simulink model "SSC17_QuanserPart2_PIDdesign"  (R2016b)
settings: Solver=ode4  StartTime=0.0  StopTime=100  FixedStep=0.01  MaxStep=2.0  RelTol=1e-3  EnableMultiTasking=on
values from neighbouring files (symbols this model uses):
  Kd = G    [UpdatedSimulinkValues-2.m]    (also in UpdatedSimulinkValuesalex1.m; part2a.m = 0.1)
  Ki = G    [UpdatedSimulinkValues-2.m]    (also in UpdatedSimulinkValuesalex1.m; part2a.m = 0.1)
  Kp = G    [UpdatedSimulinkValues-2.m]    (also in UpdatedSimulinkValuesalex1.m; part2a.m = 0.1)
settings Model: Creator=am13440  LastModifiedBy=Alex
settings DataIOCC: LimitDataPoints=on  SaveFormat=Array
settings OptimizationCC: LifeSpan=inf
settings DebuggingCC: UnderspecifiedInitializationDetection=Classic  MergeDetectMultiDrivingBlocksExec=none  SolverPrmCheckMsg=warning  StateNameClashWarn=warning  SFUnexpectedBacktrackingDiag=warning  SFNoUnconditionalDefaultTransitionDiag=warning  SFExecutionAtInitializationDiag=none
settings HardwareCC: ProdBitPerPointer=32  ProdBitPerSizeT=32  ProdBitPerPtrDiffT=32  ProdLargestAtomicFloat=None  ProdIntDivRoundTo=Undefined  ProdEndianess=Unspecified  ProdWordSize=32  ProdHWDeviceType=32-bit Generic
settings ModelReferenceCC: PropagateSignalLabelsOutOfModel=off
settings GRTTargetCC: TargetLangStandard=C89/C90 (ANSI)  GeneratePreprocessorConditionals=Disable all
settings ConfigComp: CovMetricSettings=dw  CovHtmlReporting=on  CovSaveCumulativeToWorkspaceVar=on  CovSaveSingleToWorkspaceVar=on  CovExternalEMLEnable=off  CovSFcnEnable=off

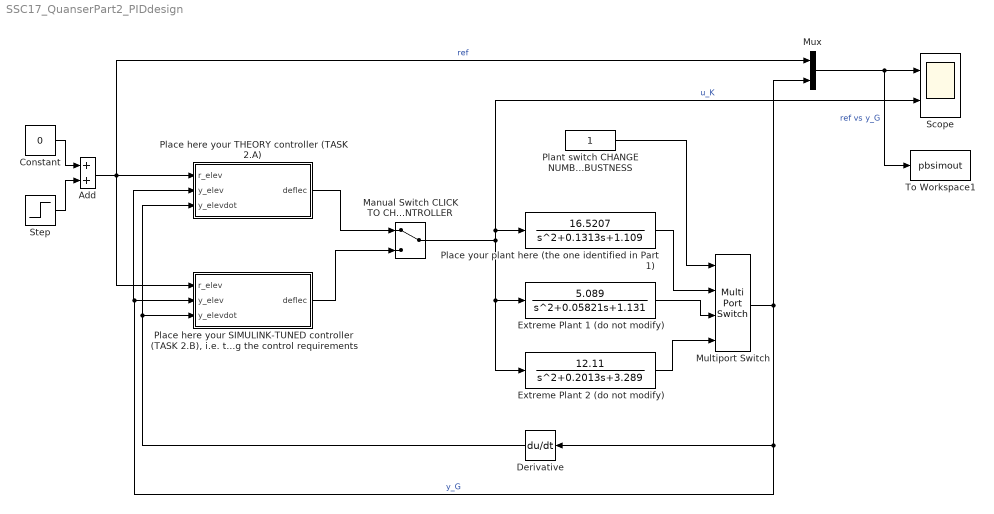
== system SSC17_QuanserPart2_PIDdesign ==
  Add : Sum
  Constant : Constant  Value=0
  Derivative : Derivative  CoefficientInTFapproximation=100
  Extreme Plant 1 (do not modify) : TransferFcn  Numerator=[5.089]  Denominator="[1  0.05821   1.131]"
  Extreme Plant 2 (do not modify) : TransferFcn  Numerator=[12.11]  Denominator="[1    0.2013   3.289]"
  Manual Switch CLICK TO CHANGE BETWEEN CONTROLLER : ManualSwitch
  Multiport Switch : MultiPortSwitch
  Mux : Mux  Inputs=2
  "Place here your SIMULINK-TUNED controller (TASK 2.B), i.e. the one satisfying the control requirements" : Subsystem
  Place here your THEORY controller (TASK 2.A) : Subsystem
  Place your plant here (the one identified in Part 1) : TransferFcn  Numerator=[16.5207]  Denominator=[1 0.1313 1.109]
  Plant switch CHANGE NUMBER [1 / 2 /  3] TO SELECT AMONG PLANTS AND TEST ROBUSTNESS : Constant
  Scope : Scope  NumInputPorts=2
  Step : Step  Time=10  SampleTime=0
  To Workspace1 : ToWorkspace  VariableName=pbsimout  SaveFormat=Timeseries  SampleTime=-1
  wires:
  Constant/1 -> Add/1
  Step/1 -> Add/2
  Add/1 -> Mux/1, Place here your THEORY controller (TASK 2.A)/1(r_elev), "Place here your SIMULINK-TUNED controller (TASK 2.B), i.e. the one satisfying the control requirements"/1(r_elev)  "ref"
  Derivative/1 -> Place here your THEORY controller (TASK 2.A)/3(y_elevdot), "Place here your SIMULINK-TUNED controller (TASK 2.B), i.e. the one satisfying the control requirements"/3(y_elevdot)
  Mux/1 -> To Workspace1/1, Scope/1  "ref vs y_G"
  Manual Switch CLICK TO CHANGE BETWEEN CONTROLLER/1 -> Scope/2, Place your plant here (the one identified in Part 1)/1, Extreme Plant 1 (do not modify)/1, Extreme Plant 2 (do not modify)/1  "u_K"
  Place here your THEORY controller (TASK 2.A)/1(deflec) -> Manual Switch CLICK TO CHANGE BETWEEN CONTROLLER/1
  "Place here your SIMULINK-TUNED controller (TASK 2.B), i.e. the one satisfying the control requirements"/1(deflec) -> Manual Switch CLICK TO CHANGE BETWEEN CONTROLLER/2
  Place your plant here (the one identified in Part 1)/1 -> Multiport Switch/2
  Extreme Plant 1 (do not modify)/1 -> Multiport Switch/3
  Extreme Plant 2 (do not modify)/1 -> Multiport Switch/4
  Multiport Switch/1 -> Place here your THEORY controller (TASK 2.A)/2(y_elev), "Place here your SIMULINK-TUNED controller (TASK 2.B), i.e. the one satisfying the control requirements"/2(y_elev), Derivative/1, Mux/2  "y_G"
  Plant switch CHANGE NUMBER [1 / 2 /  3] TO SELECT AMONG PLANTS AND TEST ROBUSTNESS/1 -> Multiport Switch/1

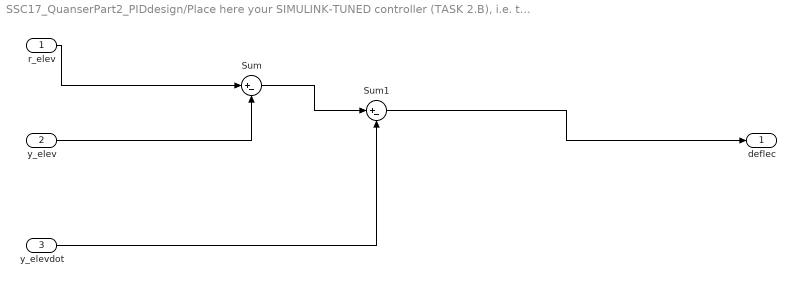
== system SSC17_QuanserPart2_PIDdesign/Place here your SIMULINK-TUNED controller (TASK 2.B), i.e. the one satisfying the control requirements ==
  r_elev : Inport
  y_elev : Inport  Port=2
  y_elevdot : Inport  Port=3
  Sum : Sum  Inputs=|+-
  Sum1 : Sum  Inputs=|+-
  deflec : Outport
  wires:
  r_elev/1 -> Sum/1
  y_elev/1 -> Sum/2
  y_elevdot/1 -> Sum1/2
  Sum/1 -> Sum1/1
  Sum1/1 -> deflec/1

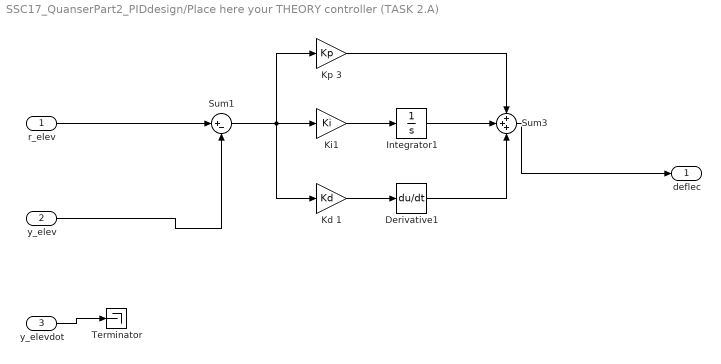
== system SSC17_QuanserPart2_PIDdesign/Place here your THEORY controller (TASK 2.A) ==
  r_elev : Inport
  y_elev : Inport  Port=2
  y_elevdot : Inport  Port=3
  Derivative1 : Derivative
  Integrator1 : Integrator
  Kd 1 : Gain  Gain=Kd
  Ki1 : Gain  Gain=Ki
  Kp 3 : Gain  Gain=Kp
  Sum1 : Sum  Inputs=|+-
  Sum3 : Sum  Inputs=+++
  Terminator : Terminator
  deflec : Outport
  wires:
  y_elev/1 -> Sum1/2
  r_elev/1 -> Sum1/1
  Sum1/1 -> Kp 3/1, Kd 1/1, Ki1/1
  Ki1/1 -> Integrator1/1
  Integrator1/1 -> Sum3/2
  Kd 1/1 -> Derivative1/1
  Derivative1/1 -> Sum3/3
  Kp 3/1 -> Sum3/1
  Sum3/1 -> deflec/1
  y_elevdot/1 -> Terminator/1
